simulink model "GreenHouseModel"  (R2015a)
settings: Solver=ode45  StartTime=0.0  StopTime=10000  RelTol=1e-3
PreLoadFcn:
  | %Density of interior air (Kg/m^3)
  | pa = 1.137;
  | %Specific Heat of Air(J/Kg.K)
  | Ca = 1005;
  | %Cover absorptivity of solar radiation
  | ac =0.1;
  | %Cover transmittance
  | tc = 0.85;
  | %Length of GreenHouse(m)
  | len = 20;
  | %Width of greenhouse(m)
  | wid = 10;
  | %Height of GreenHouse(m)[without Roof]
  | heig = 3;
  | %Roof angle from Horizontal(degrees)
  | angle = 40;
  | %Volume of greenhouse
  | Vol = len*wid*heig+0.5*wid*((width/2)*tan(angle))*len;
  | %Surface area of Greenhouse(m^2)
  | S = 2*(len*heig+wid*heig)+wid*((width/2)*tan(angle))+2*(((wid/2)/cos(angle))*len);
  | %Cover K(W/m.K)(polyethylene)
  | Kc = 0.028;
  | %Cover Thickness (m)
  | Lc = 0.03;
  | %Vertical Section of greenhouse
  | Sc = 2*(len*heig+wid*heig);
  | 
values from neighbouring files (symbols this model uses):
  Av = 2.2    [GreenHouseData.m]
  H = Vol/(len*wid)    [GreenHouseData.m]
  Hout = 60    [GreenHouseData.m]
  I = 200    [GreenHouseData.m]
  Kv = 0.7    [GreenHouseData.m]
  mairdot = 1    [GreenHouseData.m]
  Mdot = 1    [GreenHouseData.m]
  mwaterdot = 0.1    [GreenHouseData.m]
  R = 5    [GreenHouseData.m]
  rv = 0.5    [GreenHouseData.m]
  THeater = 50    [GreenHouseData.m]
  Ti = 20    [GreenHouseData.m]
  To = 10    [GreenHouseData.m]
  Twi = To    (= 10)    [GreenHouseData.m]
  Vw = 1    [GreenHouseData.m]
libraries: simulink x2, sldrtlib x1
settings Model: Creator=Aakesh Jain  LastModifiedBy=Aakesh Jain
settings DataIOCC: ExternalInput=Vol

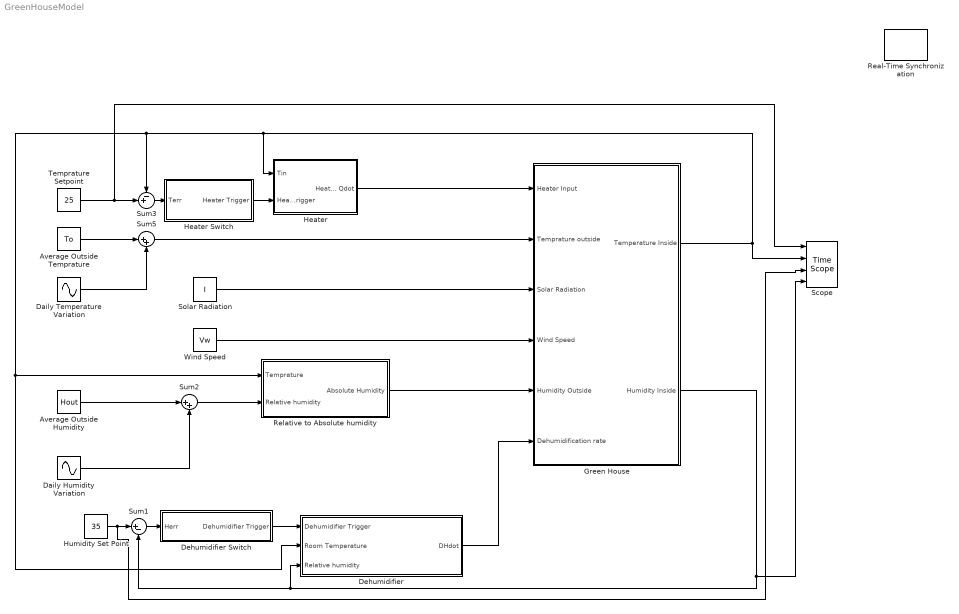
== system GreenHouseModel ==
  Average Outside Humidity : Constant  Value=Hout
  "Average Outside Temprature " : Constant  Value=To
  Daily Humidity Variation : Sin  Amplitude=5  Frequency=0.005  Phase=1.5708  SampleTime=0
  Daily Temperature Variation : Sin  Amplitude=5  SampleTime=0
  Dehumidifier : Subsystem
  Dehumidifier Switch : Subsystem
  Green House : Subsystem
  Heater : Subsystem
  Heater Switch : Subsystem
  Humidity Set Point : Constant  Value=35
  Real-Time Synchronization : sldrtlib/Real-Time Synchronization  SampleTime=0.01  MaxMissedTicks=10  ShowMissedTicks=off  YieldWhenWaiting=off
  Relative to Absolute humidity : Subsystem
  Scope : TimeScope  NumInputPorts=4
  Solar Radiation : Constant  Value=I
  Sum1 : Sum  Inputs=|+-
  Sum2 : Sum  Inputs=|++
  Sum3 : Sum  Inputs=-+|
  Sum5 : Sum  Inputs=|++
  Temprature Setpoint : Constant  Value=25
  Wind Speed : Constant  Value=Vw
  wires:
  Heater Switch/1(Heater Trigger) -> Heater/2(Heater trigger)
  Sum3/1 -> Heater Switch/1(Terr)
  "Average Outside Temprature "/1 -> Sum5/1
  Temprature Setpoint/1 -> Sum3/2, Scope/1
  Green House/1(Temperature Inside) -> Scope/2, Dehumidifier/2(Room Temperature), Relative to Absolute humidity/1(Temprature), Sum3/1, Heater/1(Tin)
  Heater/1(Heater Qdot) -> Green House/1(Heater Input)
  Sum5/1 -> Green House/2(Temprature outside)
  Wind Speed/1 -> Green House/4(Wind Speed)
  Relative to Absolute humidity/1(Absolute Humidity) -> Green House/5(Humidity Outside)
  Daily Temperature Variation/1 -> Sum5/2
  Solar Radiation/1 -> Green House/3(Solar Radiation)
  Dehumidifier Switch/1(Dehumidifier Trigger) -> Dehumidifier/1(Dehumidifier Trigger)
  Sum1/1 -> Dehumidifier Switch/1(Herr)
  Humidity Set Point/1 -> Scope/3, Sum1/1
  Dehumidifier/1(DHdot) -> Green House/6(Dehumidification rate)
  Green House/2(Humidity Inside) -> Scope/4, Sum1/2, Dehumidifier/3(Relative humidity)
  Average Outside Humidity/1 -> Sum2/1
  Sum2/1 -> Relative to Absolute humidity/2(Relative humidity)
  Daily Humidity Variation/1 -> Sum2/2

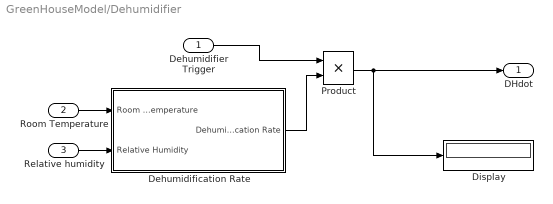
== system GreenHouseModel/Dehumidifier ==
  Dehumidifier Trigger : Inport
  Room Temperature : Inport  Port=2
  Relative humidity : Inport  Port=3
  Dehumidification Rate : Subsystem
  Display : Display
  Product : Product
  DHdot : Outport
  wires:
  Dehumidifier Trigger/1 -> Product/1
  Dehumidification Rate/1(Dehumidification Rate) -> Product/2
  Product/1 -> Display/1, DHdot/1
  Room Temperature/1 -> Dehumidification Rate/1(Room Temperature)
  Relative humidity/1 -> Dehumidification Rate/2(Relative Humidity)

== system GreenHouseModel/Dehumidifier Switch ==
  Herr : Inport
  PID Controller : simulink/Continuous/PID Controller  Controller=PID  TimeDomain=Continuous-time  SampleTime=-1  IntegratorMethod=Forward Euler  FilterMethod=Forward Euler  Form=Parallel  UseFilter=on  ControllerParametersSource=internal  P=5000  I=10  D=1  N=1  InitialConditionSource=internal  InitialConditionForIntegrator=0  InitialConditionForFilter=0  ExternalReset=none  LimitOutput=off  UpperSaturationLimit=inf  LowerSaturationLimit=-inf  LinearizeAsGain=on  AntiWindupMode=none  Kb=1  TrackingMode=off  Kt=1  PParamMin=[]  PParamMax=[]  IParamMin=[]  IParamMax=[]  DParamMin=[]  DParamMax=[]  NParamMin=[]  NParamMax=[]  KbParamMin=[]  KbParamMax=[]  KtParamMin=[]  KtParamMax=[]  POutMin=[]  POutMax=[]  IOutMin=[]  IOutMax=[]  DOutMin=[]  DOutMax=[]  NOutMin=[]  NOutMax=[]  KbOutMin=[]  KbOutMax=[]  KtOutMin=[]  KtOutMax=[]  IntegratorOutMin=[]  IntegratorOutMax=[]  FilterOutMin=[]  FilterOutMax=[]  SumOutMin=[]  SumOutMax=[]  SumI1OutMin=[]  SumI1OutMax=[]  SumI2OutMin=[]  SumI2OutMax=[]  SumI3OutMin=[]  SumI3OutMax=[]  SumDOutMin=[]  SumDOutMax=[]  SaturationOutMin=[]  SaturationOutMax=[]  IntegratorContinuousStateAttributes=''  IntegratorStateMustResolveToSignalObject=off  IntegratorRTWStateStorageClass=Auto  FilterContinuousStateAttributes=''  FilterStateMustResolveToSignalObject=off  FilterRTWStateStorageClass=Auto  DifferentiatorICPrevScaledInput=0  DifferentiatorOutMin=[]  DifferentiatorOutMax=[]
  Relay : Relay  OnSwitchValue=1  OffSwitchValue=1  ZeroCross=off
  Dehumidifier Trigger : Outport
  wires:
  Relay/1 -> Dehumidifier Trigger/1
  Herr/1 -> PID Controller/1
  PID Controller/1 -> Relay/1

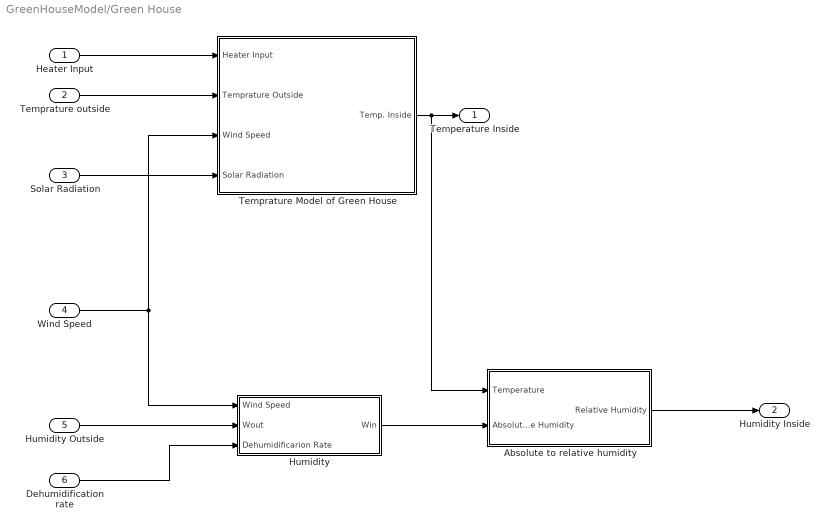
== system GreenHouseModel/Green House ==
  Heater Input : Inport
  Temprature outside : Inport  Port=2
  Solar Radiation : Inport  Port=3
  Wind Speed : Inport  Port=4
  Humidity Outside : Inport  Port=5
  Dehumidification rate : Inport  Port=6
  Absolute to relative humidity : Subsystem
  Humidity : Subsystem
  Temprature Model of Green House : Subsystem
  Temperature Inside : Outport
  Humidity Inside : Outport  Port=2
  wires:
  Temprature Model of Green House/1(Temp. Inside) -> Absolute to relative humidity/1(Temperature), Temperature Inside/1
  Heater Input/1 -> Temprature Model of Green House/1(Heater Input)
  Wind Speed/1 -> Humidity/1(Wind Speed), Temprature Model of Green House/3(Wind Speed)
  Temprature outside/1 -> Temprature Model of Green House/2(Temprature Outside)
  Solar Radiation/1 -> Temprature Model of Green House/4(Solar Radiation)
  Humidity Outside/1 -> Humidity/2(Wout)
  Humidity/1(Win) -> Absolute to relative humidity/2(Absolute Humidity)
  Absolute to relative humidity/1(Relative Humidity) -> Humidity Inside/1
  Dehumidification rate/1 -> Humidity/3(Dehumidificarion Rate)

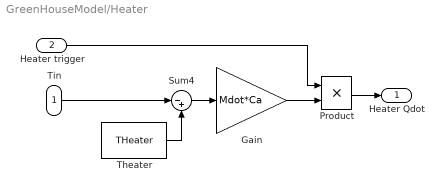
== system GreenHouseModel/Heater ==
  Tin : Inport
  Heater trigger : Inport  Port=2
  Gain : Gain  Gain=Mdot*Ca
  Product : Product
  Sum4 : Sum  Inputs=|-+
  Theater : Constant  Value=THeater
  Heater Qdot : Outport
  wires:
  Theater/1 -> Sum4/2
  Product/1 -> Heater Qdot/1
  Gain/1 -> Product/2
  Heater trigger/1 -> Product/1
  Sum4/1 -> Gain/1
  Tin/1 -> Sum4/1

== system GreenHouseModel/Heater Switch ==
  Terr : Inport
  PID Controller : simulink/Continuous/PID Controller  Controller=PID  TimeDomain=Continuous-time  SampleTime=-1  IntegratorMethod=Forward Euler  FilterMethod=Forward Euler  Form=Parallel  UseFilter=on  ControllerParametersSource=internal  P=20  I=2  D=1000  N=1  InitialConditionSource=internal  InitialConditionForIntegrator=0  InitialConditionForFilter=0  ExternalReset=none  LimitOutput=off  UpperSaturationLimit=inf  LowerSaturationLimit=-inf  LinearizeAsGain=on  AntiWindupMode=none  Kb=1  TrackingMode=off  Kt=1  PParamMin=[]  PParamMax=[]  IParamMin=[]  IParamMax=[]  DParamMin=[]  DParamMax=[]  NParamMin=[]  NParamMax=[]  KbParamMin=[]  KbParamMax=[]  KtParamMin=[]  KtParamMax=[]  POutMin=[]  POutMax=[]  IOutMin=[]  IOutMax=[]  DOutMin=[]  DOutMax=[]  NOutMin=[]  NOutMax=[]  KbOutMin=[]  KbOutMax=[]  KtOutMin=[]  KtOutMax=[]  IntegratorOutMin=[]  IntegratorOutMax=[]  FilterOutMin=[]  FilterOutMax=[]  SumOutMin=[]  SumOutMax=[]  SumI1OutMin=[]  SumI1OutMax=[]  SumI2OutMin=[]  SumI2OutMax=[]  SumI3OutMin=[]  SumI3OutMax=[]  SumDOutMin=[]  SumDOutMax=[]  SaturationOutMin=[]  SaturationOutMax=[]  IntegratorContinuousStateAttributes=''  IntegratorStateMustResolveToSignalObject=off  IntegratorRTWStateStorageClass=Auto  FilterContinuousStateAttributes=''  FilterStateMustResolveToSignalObject=off  FilterRTWStateStorageClass=Auto  DifferentiatorICPrevScaledInput=0  DifferentiatorOutMin=[]  DifferentiatorOutMax=[]
  Relay : Relay  OnSwitchValue=0  OffSwitchValue=-0.1  ZeroCross=off
  Heater Trigger : Outport
  wires:
  Relay/1 -> Heater Trigger/1
  Terr/1 -> PID Controller/1
  PID Controller/1 -> Relay/1

== system GreenHouseModel/Relative to Absolute humidity ==
  Temprature : Inport
  Relative humidity : Inport  Port=2
  Product : Product
  Temprature function : Fcn  Expr=((0.004055)+(0.0001152*u)+0.00002167*u^2)/100
  Absolute Humidity : Outport
  wires:
  Temprature/1 -> Temprature function/1
  Product/1 -> Absolute Humidity/1
  Relative humidity/1 -> Product/2
  Temprature function/1 -> Product/1

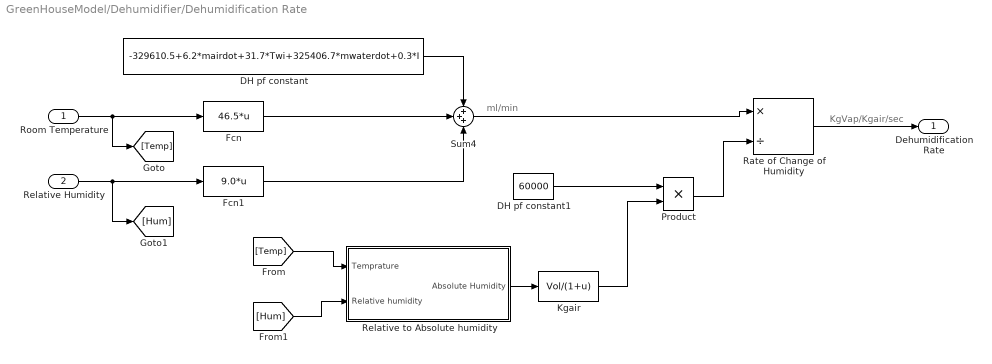
== system GreenHouseModel/Dehumidifier/Dehumidification Rate ==
  note: KgVap/Kgair/sec
  note: ml/min
  Room Temperature : Inport
  Relative Humidity : Inport  Port=2
  DH pf constant : Constant  Value=-329610.5+6.2*mairdot+31.7*Twi+325406.7*mwaterdot+0.3*I
  DH pf constant1 : Constant  Value=60000
  Fcn : Fcn  Expr=46.5*u
  Fcn1 : Fcn  Expr=9.0*u
  Kgair : Fcn  Expr=Vol/(1+u)
  Product : Product
  Rate of Change of Humidity : Product  Inputs=*/
  Relative to Absolute humidity : Subsystem
  Sum4 : Sum  Inputs=+++
  Dehumidification Rate : Outport
  wires:
  Relative Humidity/1 -> [Hum], Fcn1/1
  Room Temperature/1 -> [Temp], Fcn/1
  Sum4/1 -> Rate of Change of Humidity/1
  DH pf constant/1 -> Sum4/1
  Fcn/1 -> Sum4/2
  Fcn1/1 -> Sum4/3
  Relative to Absolute humidity/1(Absolute Humidity) -> Kgair/1
  [Temp] -> Relative to Absolute humidity/1(Temprature)
  [Hum] -> Relative to Absolute humidity/2(Relative humidity)
  Kgair/1 -> Product/2
  Rate of Change of Humidity/1 -> Dehumidification Rate/1
  DH pf constant1/1 -> Product/1
  Product/1 -> Rate of Change of Humidity/2

== system GreenHouseModel/Green House/Absolute to relative humidity ==
  Temperature : Inport
  Absolute Humidity : Inport  Port=2
  Rate of Change of Humidity : Product  Inputs=*/
  Temprature function : Fcn  Expr=((0.004055)+(0.0001152*u)+0.00002167*u^2)/100
  Relative Humidity : Outport
  wires:
  Temprature function/1 -> Rate of Change of Humidity/2
  Absolute Humidity/1 -> Rate of Change of Humidity/1
  Rate of Change of Humidity/1 -> Relative Humidity/1
  Temperature/1 -> Temprature function/1

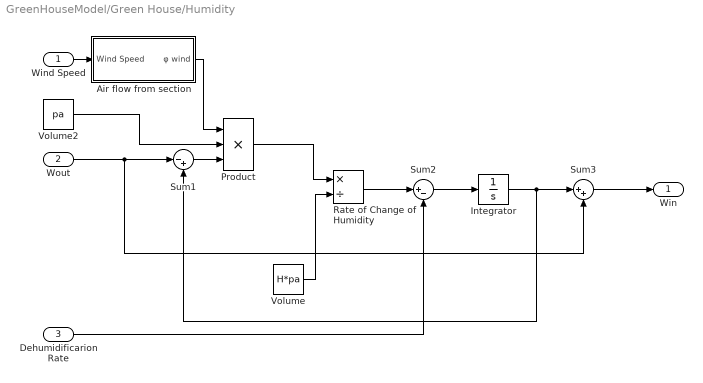
== system GreenHouseModel/Green House/Humidity ==
  Wind Speed : Inport
  Wout : Inport  Port=2
  Dehumidificarion Rate : Inport  Port=3
  Air flow from section : Subsystem
  Integrator : Integrator
  Product : Product  Inputs=3
  Rate of Change of Humidity : Product  Inputs=*/
  Sum1 : Sum  Inputs=|-+
  Sum2 : Sum  Inputs=|+-
  Sum3 : Sum  Inputs=|++
  Volume : Constant  Value=H*pa
  Volume2 : Constant  Value=pa
  Win : Outport
  wires:
  Air flow from section/1(φ wind) -> Product/1
  Sum1/1 -> Product/3
  Volume/1 -> Rate of Change of Humidity/2
  Wout/1 -> Sum3/2, Sum1/1
  Wind Speed/1 -> Air flow from section/1(Wind Speed)
  Integrator/1 -> Sum3/1, Sum1/2
  Volume2/1 -> Product/2
  Product/1 -> Rate of Change of Humidity/1
  Dehumidificarion Rate/1 -> Sum2/2
  Rate of Change of Humidity/1 -> Sum2/1
  Sum2/1 -> Integrator/1
  Sum3/1 -> Win/1

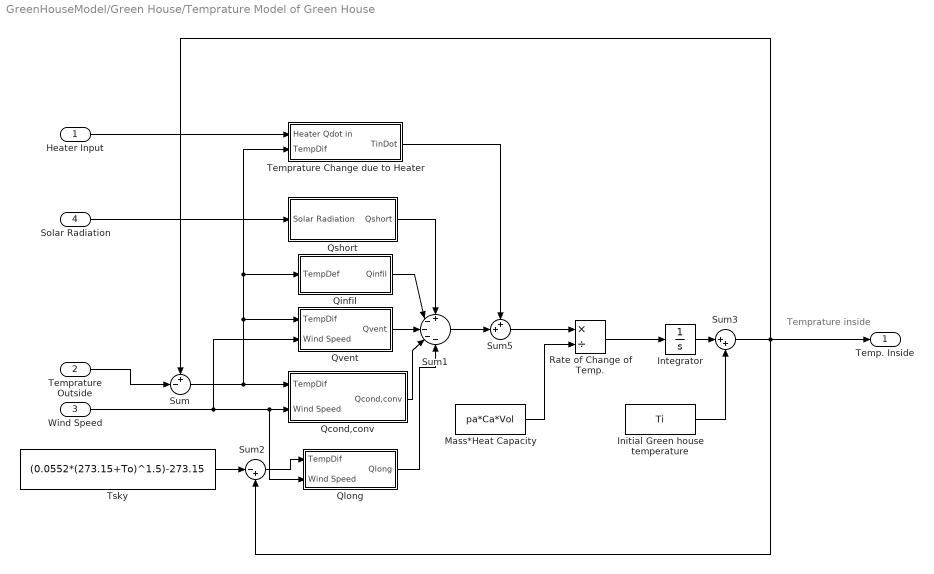
== system GreenHouseModel/Green House/Temprature Model of Green House ==
  note: Temprature
      | inside
  Heater Input : Inport
  Temprature Outside : Inport  Port=2
  Wind Speed : Inport  Port=3
  Solar Radiation : Inport  Port=4
  Initial Green house temperature : Constant  Value=Ti
  Integrator : Integrator
  Mass*Heat Capacity : Constant  Value=pa*Ca*Vol
  Qcond,conv : Subsystem
  Qinfil : Subsystem
  Qlong : Subsystem
  Qshort : Subsystem
  Qvent : Subsystem
  Rate of Change of Temp. : Product  Inputs=*/
  Sum : Sum  Inputs=+-|
  Sum1 : Sum  Inputs=+----
  Sum2 : Sum  Inputs=|-+
  Sum3 : Sum  Inputs=|++
  Sum5 : Sum  Inputs=++|
  Temprature Change due to Heater : Subsystem
  Tsky : Constant  Value=(0.0552*(273.15+To)^1.5)-273.15
  Temp. Inside : Outport
  wires:
  Sum2/1 -> Qlong/1(TempDif)
  Mass*Heat Capacity/1 -> Rate of Change of Temp./2
  Sum/1 -> Temprature Change due to Heater/2(TempDif), Qinfil/1("TempDef "), Qvent/1(TempDif), Qcond,conv/1("TempDif ")
  Qshort/1(Qshort) -> Sum1/1
  Heater Input/1 -> Temprature Change due to Heater/1(Heater Qdot in)
  Temprature Outside/1 -> Sum/2
  Rate of Change of Temp./1 -> Integrator/1
  Qinfil/1("Qinfil ") -> Sum1/2
  Tsky/1 -> Sum2/1
  Wind Speed/1 -> Qvent/2(Wind Speed), Qlong/2(Wind Speed), Qcond,conv/2(Wind Speed)
  Integrator/1 -> Sum3/1
  Qlong/1(Qlong) -> Sum1/5
  Qcond,conv/1(Qcond,conv) -> Sum1/4
  Solar Radiation/1 -> Qshort/1(Solar Radiation)
  Qvent/1(Qvent) -> Sum1/3
  Sum3/1 -> Sum2/2, Temp. Inside/1, Sum/1
  Initial Green house temperature/1 -> Sum3/2
  Sum1/1 -> Sum5/2
  Sum5/1 -> Rate of Change of Temp./1
  Temprature Change due to Heater/1(TinDot) -> Sum5/1

== system GreenHouseModel/Dehumidifier/Dehumidification Rate/Relative to Absolute humidity ==
  Temprature : Inport
  Relative humidity : Inport  Port=2
  Product : Product
  Temprature function : Fcn  Expr=((0.004055)+(0.0001152*u)+0.00002167*u^2)/100
  Absolute Humidity : Outport
  wires:
  Temprature/1 -> Temprature function/1
  Product/1 -> Absolute Humidity/1
  Relative humidity/1 -> Product/2
  Temprature function/1 -> Product/1

== system GreenHouseModel/Green House/Humidity/Air flow from section ==
  Wind Speed : Inport
  Product : Product
  Vertical Section : Constant  Value=Av/Sc
  φ wind : Outport
  wires:
  Wind Speed/1 -> Product/1
  Product/1 -> φ wind/1
  Vertical Section/1 -> Product/2

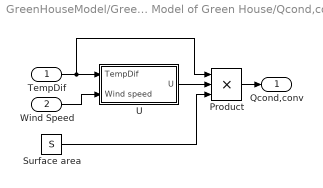
== system GreenHouseModel/Green House/Temprature Model of Green House/Qcond,conv ==
  "TempDif " : Inport
  Wind Speed : Inport  Port=2
  Product : Product  Inputs=3
  Surface area : Constant  Value=S
  "U " : Subsystem
  Qcond,conv : Outport
  wires:
  Product/1 -> Qcond,conv/1
  "TempDif "/1 -> Product/1, "U "/1("TempDif ")
  Surface area/1 -> Product/3
  "U "/1("U ") -> Product/2
  Wind Speed/1 -> "U "/2(Wind speed)

== system GreenHouseModel/Green House/Temprature Model of Green House/Qinfil ==
  "TempDef " : Inport
  "Constant " : Constant  Value=pa*Ca*R/3600
  Product : Product
  "Qinfil " : Outport
  wires:
  "Constant "/1 -> Product/1
  Product/1 -> "Qinfil "/1
  "TempDef "/1 -> Product/2

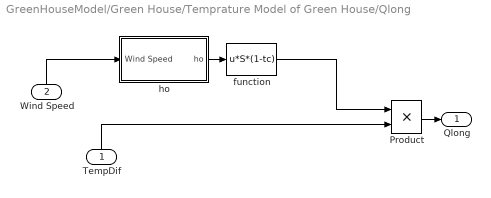
== system GreenHouseModel/Green House/Temprature Model of Green House/Qlong ==
  TempDif : Inport
  Wind Speed : Inport  Port=2
  " function" : Fcn  Expr=u*S*(1-tc)
  Product : Product
  ho : Subsystem
  Qlong : Outport
  wires:
  TempDif/1 -> Product/2
  " function"/1 -> Product/1
  Product/1 -> Qlong/1
  Wind Speed/1 -> ho/1(Wind Speed)
  ho/1(ho) -> " function"/1

== system GreenHouseModel/Green House/Temprature Model of Green House/Qshort ==
  Solar Radiation : Inport
  Constant : Constant  Value=ac*tc*S
  Product : Product
  Qshort : Outport
  wires:
  Solar Radiation/1 -> Product/2
  Product/1 -> Qshort/1
  Constant/1 -> Product/1

== system GreenHouseModel/Green House/Temprature Model of Green House/Qvent ==
  TempDif : Inport
  Wind Speed : Inport  Port=2
  Constant : Constant  Value=rv*Kv*Av*pa*Ca
  Product : Product  Inputs=3
  Qvent : Outport
  wires:
  TempDif/1 -> Product/2
  Wind Speed/1 -> Product/3
  Product/1 -> Qvent/1
  Constant/1 -> Product/1

== system GreenHouseModel/Green House/Temprature Model of Green House/Temprature Change due to Heater ==
  Heater Qdot in : Inport
  TempDif : Inport  Port=2
  Gain1 : Gain  Gain=1/Kc
  Sum5 : Sum  Inputs=|+-
  TinDot : Outport
  wires:
  TempDif/1 -> Gain1/1
  Heater Qdot in/1 -> Sum5/1
  Sum5/1 -> TinDot/1
  Gain1/1 -> Sum5/2

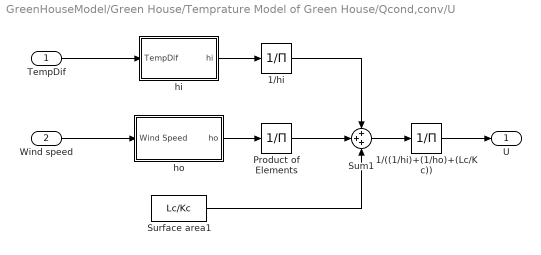
== system GreenHouseModel/Green House/Temprature Model of Green House/Qcond,conv/U  ==
  "TempDif " : Inport
  Wind speed : Inport  Port=2
  1/((1/hi)+(1/ho)+(Lc/Kc)) : Product  Inputs=/
  1/hi : Product  Inputs=/
  Product of Elements : Product  Inputs=/
  Sum1 : Sum  Inputs=+++
  Surface area1 : Constant  Value=Lc/Kc
  hi : Subsystem
  ho : Subsystem
  "U " : Outport
  wires:
  "TempDif "/1 -> hi/1("TempDif ")
  hi/1("hi ") -> 1/hi/1
  1/((1/hi)+(1/ho)+(Lc/Kc))/1 -> "U "/1
  Sum1/1 -> 1/((1/hi)+(1/ho)+(Lc/Kc))/1
  1/hi/1 -> Sum1/1
  Wind speed/1 -> ho/1(Wind Speed)
  ho/1(ho) -> Product of Elements/1
  Product of Elements/1 -> Sum1/2
  Surface area1/1 -> Sum1/3

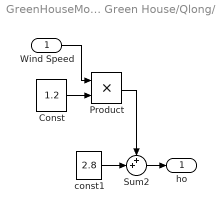
== system GreenHouseModel/Green House/Temprature Model of Green House/Qlong/ho ==
  Wind Speed : Inport
  Const : Constant  Value=1.2
  Product : Product
  Sum2 : Sum  Inputs=++|
  const1 : Constant  Value=2.8
  ho : Outport
  wires:
  Sum2/1 -> ho/1
  Wind Speed/1 -> Product/1
  Const/1 -> Product/2
  Product/1 -> Sum2/1
  const1/1 -> Sum2/2

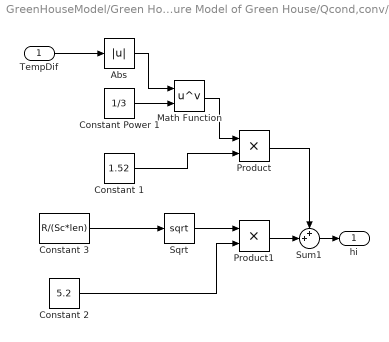
== system GreenHouseModel/Green House/Temprature Model of Green House/Qcond,conv/U /hi ==
  "TempDif " : Inport
  Abs : Abs
  Constant 1 : Constant  Value=1.52
  Constant 2 : Constant  Value=5.2
  Constant 3 : Constant  Value=R/(Sc*len)
  Constant Power 1 : Constant  Value=1/3
  Math Function : Math  Operator=pow  SaturateOnIntegerOverflow=on
  Product : Product
  Product1 : Product
  Sqrt : Sqrt  SaturateOnIntegerOverflow=on
  Sum1 : Sum  Inputs=++|
  "hi " : Outport
  wires:
  Product1/1 -> Sum1/2
  Constant 2/1 -> Product1/2
  Sum1/1 -> "hi "/1
  Math Function/1 -> Product/1
  Constant Power 1/1 -> Math Function/2
  Product/1 -> Sum1/1
  "TempDif "/1 -> Abs/1
  Constant 1/1 -> Product/2
  Constant 3/1 -> Sqrt/1
  Abs/1 -> Math Function/1
  Sqrt/1 -> Product1/1

== system GreenHouseModel/Green House/Temprature Model of Green House/Qcond,conv/U /ho ==
  Wind Speed : Inport
  Const : Constant  Value=1.2
  Product : Product
  Sum2 : Sum  Inputs=++|
  const1 : Constant  Value=2.8
  ho : Outport
  wires:
  Sum2/1 -> ho/1
  Wind Speed/1 -> Product/1
  Const/1 -> Product/2
  Product/1 -> Sum2/1
  const1/1 -> Sum2/2
